simulink model "inverse_dynamics"  (R2017b)
settings: Solver=FixedStepAuto  StartTime=0.0  StopTime=100  FixedStep=0.2  RelTol=1e-3
values from neighbouring files (symbols this model uses):
  kd = 5    [PD_gravity_compensation_init.m]    (also in inverse_dynamics_init.m)
  kp = 2    [PD_gravity_compensation_init.m]    (also in inverse_dynamics_init.m = 3)
  q_desired = [pi/4,3*pi/4,0,3*pi/4,-pi/4,-3*pi/4]    [PD_gravity_compensation_init.m]    (also in inverse_dynamics_init.m; robot_initial_config.m = p560.ikine6s(TTCP_World_desired))
  q_initial = qz    [PD_gravity_compensation_init.m]    (also in inverse_dynamics_init.m)
  qd_lower_sat_limit = -5    [PD_gravity_compensation_init.m]    (also in inverse_dynamics_init.m)
  qd_upper_sat_limit = 5    [PD_gravity_compensation_init.m]    (also in inverse_dynamics_init.m)
  tmax = 5    [inverse_dynamics_init.m]
  ts = 0.2    [inverse_dynamics_init.m]
undefined symbols (not defined in the file or in its folder): p560, q, qd, qdd, slcoulomb
libraries: roblocks x1
settings Model: Creator=albertllebariafabrias  LastModifiedBy=albertllebariafabrias

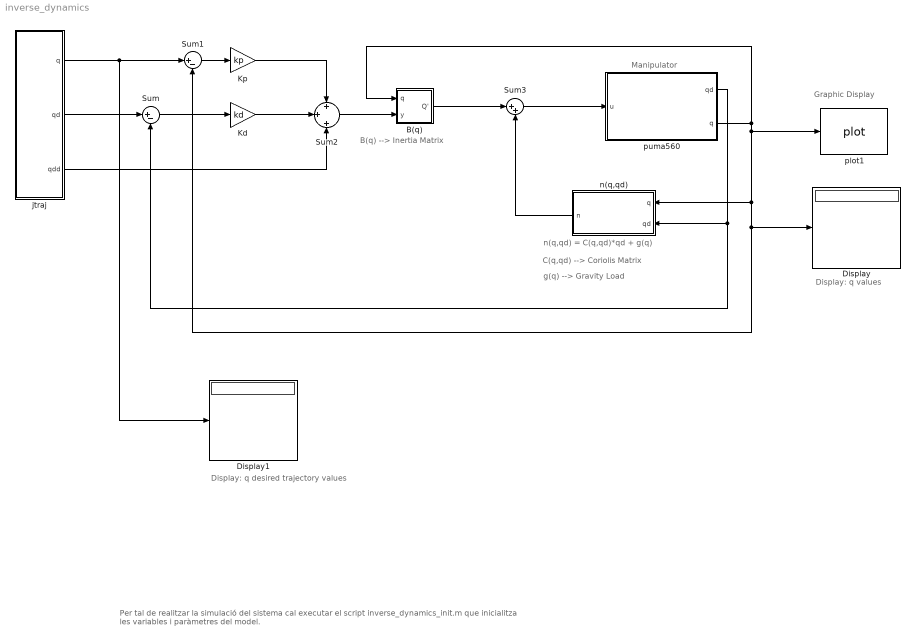
== system inverse_dynamics ==
  note: Per tal de realitzar la simulació del sistema cal executar el script inverse_dynamics_init.m que inicialitza les variables i paràmetres del model.
  note: Graphic Display
  note: Display: q values
  note: Display: q desired trajectory values
  note: n(q,qd) = C(q,qd)*qd + g(q)
  note: B(q) --> Inertia Matrix
  note: C(q,qd) --> Coriolis Matrix
  note: g(q) --> Gravity Load
  note: Manipulator
  B(q) : Subsystem
  Display : Display
  Display1 : Display
  Kd : Gain  Gain=kd
  Kp : Gain  Gain=kp
  Sum : Sum  Inputs=|+-
  Sum1 : Sum  Inputs=|+-
  Sum2 : Sum  Inputs=+|+|+
  Sum3 : Sum  Inputs=|++
  jtraj : Subsystem  AncestorBlock=roblocks/Toolbox/jtraj  mask{q0=q_initial, qf=q_desired, tmax=tmax, ts=ts}
      mask prompts: tmax "tmax (s)"; ts "ts (s)"
      mask help: Joint interpolated trajectory.
      mask init:
      | n = length(q0);
      | if length(q0) ~= length(qf) ,
      |  error('q0 and qf must be same length')
      | end
      | t=[0:100]'/100*tmax;
      | [q,qd,qdd] = jtraj(q0, qf, t);
      mask Help:
      | Generate quintic polynomial to move from initial to final joint angles as specified.  Initial and final velocity are assumed to be zero.
      | 
      | <b>Parameters::</b>
      | 
      | q0 (1xN) initial joint coordinates
      | qf (1xN) final joint coordinates
      | tmax (1x1) the time for the trajectory to complete
      | 
      | Initial and final velocity are assumed to be zero.
      | 
      | <b>Outputs::</b>
      | 
      | q (1xN) vector of joint coordinates at current simulation time
      | qd (1xN) vector of joint coordinate velocity at current simulation time
      | qdd (1xN) vector of joint coordinate acceleration at current simulation time
      | 
      | <b>Notes::</b>
      | 
      | - If simulation time exceeds tmax then q is clipped to qf.
      | - A wrapper on the Toolbox function jtraj.
      | - The piecewise constant output of jtraj is interpolated to the current
      |   simulation time.
      mask Display:
      | port_label('output', 1, 'q')
      | port_label('output', 2, 'qd')
      | port_label('output', 3, 'qdd')
  "n(q,qd) " : Subsystem
  plot1 : roblocks/Arm/plot  robot=p560  fps=fps  holdplot=on
  puma560 : Subsystem
  wires:
  puma560/2(q) -> Sum1/2, Display/1, "n(q,qd) "/1(q), plot1/1, B(q)/1("q ")
  jtraj/2(qd) -> Sum/1
  Sum/1 -> Kd/1
  Kd/1 -> Sum2/2
  jtraj/3(qdd) -> Sum2/3
  Sum3/1 -> puma560/1(u)
  puma560/1(qd) -> Sum/2, "n(q,qd) "/2("qd ")
  B(q)/1(Q') -> Sum3/1
  Sum2/1 -> B(q)/2(y)
  "n(q,qd) "/1(n) -> Sum3/2
  Kp/1 -> Sum2/1
  Sum1/1 -> Kp/1
  jtraj/1(q) -> Display1/1, Sum1/1

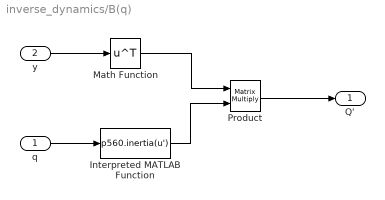
== system inverse_dynamics/B(q) ==
  "q " : Inport
  y : Inport  Port=2
  Interpreted MATLAB Function : MATLABFcn  MATLABFcn=p560.inertia(u')  Output1D=off
  Math Function : Math  Operator=transpose  SaturateOnIntegerOverflow=on
  Product : Product  Multiplication=Matrix(*)
  Q' : Outport
  wires:
  "q "/1 -> Interpreted MATLAB Function/1
  Interpreted MATLAB Function/1 -> Product/2
  y/1 -> Math Function/1
  Math Function/1 -> Product/1
  Product/1 -> Q'/1

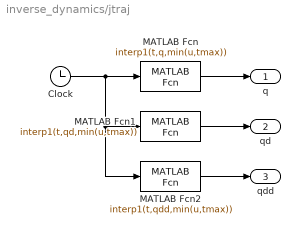
== system inverse_dynamics/jtraj ==
  Clock : Clock
  MATLAB Fcn : MATLABFcn  MATLABFcn=interp1(t,q,min(u,tmax))  OutputDimensions=n  SampleTime=ts
  MATLAB Fcn1 : MATLABFcn  MATLABFcn=interp1(t,qd,min(u,tmax))  OutputDimensions=n  SampleTime=ts
  MATLAB Fcn2 : MATLABFcn  MATLABFcn=interp1(t,qdd,min(u,tmax))  OutputDimensions=n  SampleTime=ts
  q : Outport
  qd : Outport  Port=2
  qdd : Outport  Port=3
  wires:
  MATLAB Fcn/1 -> q/1
  MATLAB Fcn1/1 -> qd/1
  Clock/1 -> MATLAB Fcn/1, MATLAB Fcn1/1, MATLAB Fcn2/1
  MATLAB Fcn2/1 -> qdd/1

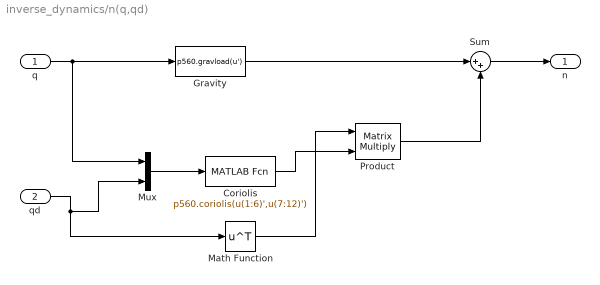
== system inverse_dynamics/n(q,qd)  ==
  q : Inport
  "qd " : Inport  Port=2
  " Coriolis" : MATLABFcn  MATLABFcn=p560.coriolis(u(1:6)',u(7:12)')  OutputDimensions=[6,6]  Output1D=off
  " Gravity " : MATLABFcn  MATLABFcn=p560.gravload(u')  Output1D=off
  Math Function : Math  Operator=transpose  SaturateOnIntegerOverflow=on
  Mux : Mux  Inputs=2
  Product : Product  Multiplication=Matrix(*)
  Sum : Sum  Inputs=|++
  n : Outport
  wires:
  " Gravity "/1 -> Sum/1
  Sum/1 -> n/1
  Math Function/1 -> Product/1
  Product/1 -> Sum/2
  q/1 -> Mux/1, " Gravity "/1
  "qd "/1 -> Mux/2, Math Function/1
  " Coriolis"/1 -> Product/2
  Mux/1 -> " Coriolis"/1

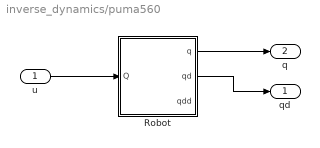
== system inverse_dynamics/puma560 ==
  u : Inport
  Robot : Subsystem  AncestorBlock=roblocks/Arm/Robot  mask{robot=p560, q0=[0,0,0,0,0,0]}
      mask prompts: robot "Robot object"; q0 "Initial state"
      mask help: Rigid-body dynamic model of robot.
      mask init:
      | if isa(robot, 'SerialLink')
      |     rname = robot.name;
      |     %fprintf('**robot name is %s\n', rname);
      | else
      |     rname = '';
      |     n = 0
      | end
      mask Help:
      | Simulates the forward (direct) rigid-body dynamics of the robot described
      | by the given robot object.  For given applied joint torque/force it computes
      | the instaneous joint coordinates, velocities and acclerations.
      | 
      | 
      | <b>Parameters::</b>
      | 
      | robot (SerialLink) a dynamic model of an N-link serial link manipulator
      | q0 (1xN)  Initial joint coordinates
      | 
      | <b>Inputs::</b>
      | 
      | Q (1xN) the generalized joint force (torque or force) required to achieve
      | the motion state (q, qd, qdd).
      | 
      | <b>Outputs::</b>
      | 
      | q (1xN) joint coordinates
      | qd (1xN) joint coordinate velocity
      | qdd (1xN) joint coordinate acceleration
      | 
      | 
      | <b>Notes::</b>
      | 
      | - Required to simulate robot rigid body motion.
      | - Implemented using the recursive Newton-Euler scheme (RNE).
      | - A wrapper for the Toolbox method accel() which in turn depends on the
      |   method rne().
      mask Display:
      | port_label('input', 1, 'Q')
      | port_label('output', 1, 'q')
      | port_label('output', 2, 'qd')
      | port_label('output', 3, 'qdd')
      | text(0.1, 0.9,  rname, 'horizontalAlignment', 'left')
  qd : Outport
  q : Outport  Port=2
  wires:
  u/1 -> Robot/1(Q)
  Robot/1(q) -> q/1
  Robot/2(qd) -> qd/1

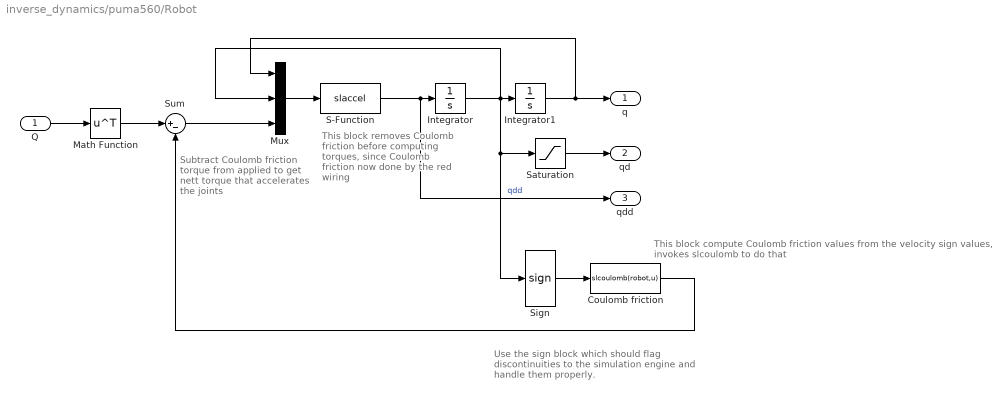
== system inverse_dynamics/puma560/Robot ==
  note: This block removes Coulomb friction before computing torques, since Coulomb friction now done by the red wiring
  note: Subtract Coulomb friction torque from applied to get nett torque that accelerates the joints
  note: This block compute Coulomb friction values from the velocity sign values, invokes slcoulomb to do that
  note: Use the sign block which should flag discontinuities to the simulation engine and
      | handle them properly.
  Q : Inport
  Coulomb friction : MATLABFcn  MATLABFcn=slcoulomb(robot,u)  OutputDimensions=[robot.n 1]  Output1D=off
  Integrator : Integrator
  Integrator1 : Integrator  InitialCondition=q0
  Math Function : Math  Operator=transpose  SaturateOnIntegerOverflow=on
  Mux : Mux  Inputs=3
  S-Function : S-Function  FunctionName=slaccel  Parameters=robot.nofriction()  SFunctionDeploymentMode=off  EnableBusSupport=off
  Saturation : Saturate  UpperLimit=qd_upper_sat_limit  LowerLimit=qd_lower_sat_limit  ZeroCross=off
  Sign : Signum
  Sum : Sum  Inputs=|+-
  q : Outport
  qd : Outport  Port=2
  qdd : Outport  Port=3
  wires:
  S-Function/1 -> qdd/1, Integrator/1  "qdd"
  Mux/1 -> S-Function/1
  Integrator/1 -> Sign/1, Saturation/1, Integrator1/1, Mux/2
  Integrator1/1 -> q/1, Mux/1
  Q/1 -> Math Function/1
  Sum/1 -> Mux/3
  Coulomb friction/1 -> Sum/2
  Sign/1 -> Coulomb friction/1
  Saturation/1 -> qd/1
  Math Function/1 -> Sum/1
